simulink model "DWmodel"  (R2025a)
settings: Solver=daessc  StartTime=0.0  StopTime=inf  MaxStep=.5  RelTol=1e-3  AbsTol=1e-3
PreLoadFcn:
  | DWmodel_ini
values from neighbouring files (symbols this model uses):
  basinArea = 0.2    [DWmodel_ini.m]
  heaterPower = 1800    [DWmodel_ini.m]
  inletPipeDia = 0.025    [DWmodel_ini.m]
  inletPipeEffLen = 2    [DWmodel_ini.m]
  lpmLeakageFlow = 0.001    [DWmodel_ini.m]
  machineHeight = 1.5    [DWmodel_ini.m]
  maxBasinLiqLevel = 0.10    (= 0.1)    [DWmodel_ini.m]
  maxBasinLiqTemp = 350    [DWmodel_ini.m]
  minBasinLiqLevel = 0.04    [DWmodel_ini.m]
  minBasinLiqTemp = 305    [DWmodel_ini.m]
  motorPower = 500    [DWmodel_ini.m]
  motorSpeed = 500    [DWmodel_ini.m]
  outletPipeDia = 0.025    [DWmodel_ini.m]
  outletPipeEffLen = 2    [DWmodel_ini.m]
  powerWashCycle = 500    [DWmodel_ini.m]
  pumpOutletDia = 0.025    [DWmodel_ini.m]
libraries: fl_lib x15, nesl_utility x8, simulink x7, SimscapeFluids_lib x3
CloseFcn:
  | try,close(h_DishwasherFaultAnalysis),end
  | clear h_DishwasherFaultAnalysis
  | 
  | clear ambient basinArea machineHeight
  | clear iniBasinLiqLevel maxBasinLiqTemp minBasinLiqTemp
  | clear maxBasinLiqLevel minBasinLiqLevel lpmLeakageFlow
  | clear motorPower motorSpeed heaterPower powerWashCycle
  | clear outletPipeEffLen outletPipeDia inletPipeEffLen inletPipeDia
  | clear pumpOutletDia pumpCapacity pumpHead pumpBrakePower pumpShaftSpeed
  | clear simlog_DishwasherFaultAnalysis tout
Description:
  | Dishwasher Fault Analysis
settings Model: Creator=The MathWorks, Inc.  LastModifiedBy=DR53SF
settings SolverCC: AutoScaleAbsTol=off  MaxConsecutiveMinStep=5  ZeroCrossAlgorithm=Adaptive  AlgebraicLoopSolver=TrustRegion  MaxZcPerStep=1.0
settings DataIOCC: SaveTime=off  ReturnWorkspaceOutputs=off
settings DebuggingCC: IgnoredZcDiagnostic=none  UnconnectedInputMsg=warning  UnconnectedOutputMsg=warning  UnconnectedLineMsg=warning  SymbolicDimsDataTypeCodeGenerationDiagnostic=none
settings ModelReferenceCC: EnableRefExpFcnMdlSchedulingChecks=on
settings SFSimCC: CustomCodeUndefinedFunction=UseInterfaceOnly
settings RTWCC: GPUComputeCapability=3.5  DLArmComputeVersion=19.05
settings SimscapeCC: SimscapeNominalValues="[{\"value\":\"1\",\"unit\":\"A\"},{\"value\":\"1\",\"unit\":\"bar\"},{\"value\":\"1\",\"unit\":\"cm^2\"},{\"value\":\"1\",\"unit\":\"cm^3/s\"},{\"value\":\"1\",\"unit\":\"kJ/kg\"},{\"value\":\"1\",\"unit\":\"kW\"},{\"value\":\"1\",\"unit\":\"l\"},{\"value\":\"1\",\"unit\":\"N\"},{\"value\":\"1\",\"unit\":\"N*m\"},{\"value\":\"1\",\"unit\":\"V\"},{\"value\":\"1e-2\",\"unit\":\"m\"}]"  SimscapeLogType=all  SimscapeLogSimulationStatistics=on  SimscapeLogName=simlog_DishwasherFaultAnalysis  SimscapeLogDataHistory=100000.0

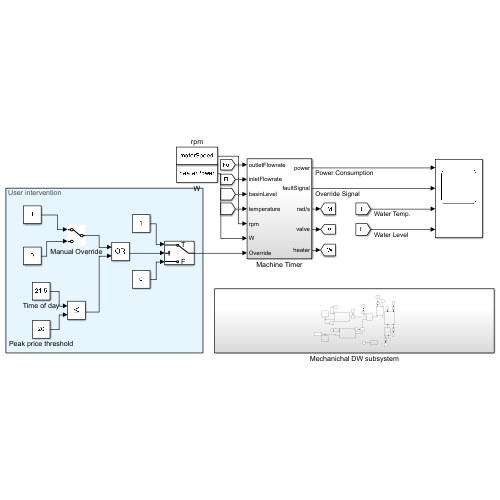
[thumbnail: Simulink's stored preview of the top-level diagram]
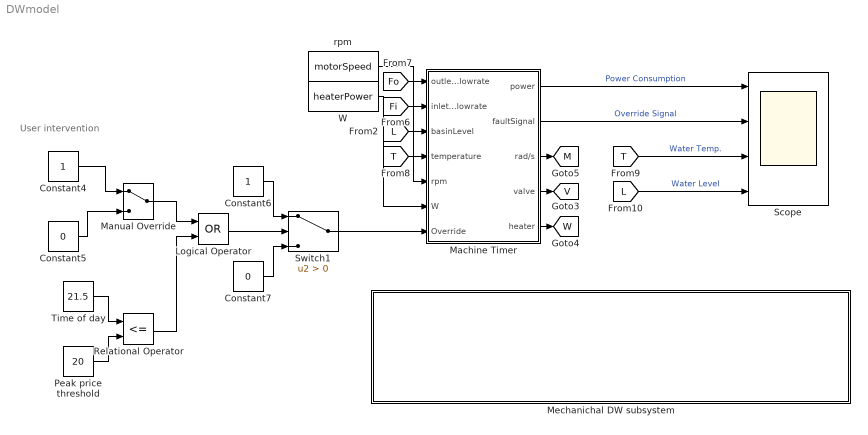
== system DWmodel ==
  note: User intervention
  Constant4 : Constant
  Constant5 : Constant  Value=0
  Constant6 : Constant
  Constant7 : Constant  Value=0
  Logical Operator : Logic  Operator=OR  AllPortsSameDT=off  OutDataTypeStr=boolean
  Machine Timer : Subsystem
  Manual Override : ManualSwitch
  Mechanichal DW subsystem : Subsystem
  Peak price threshold : Constant  Value=20
  Relational Operator : RelationalOperator  Operator=<=  OutDataTypeStr=boolean  RndMeth=Simplest  InputSameDT=off
  Scope : Scope  NumInputPorts=4
      settings: ActiveDisplayYMinimum=-348.81952121815567  ActiveDisplayYMaximum=3139.3756909634017
  Switch1 : Switch  Criteria=u2 > Threshold  SaturateOnIntegerOverflow=off  InputSameDT=off
  Time of day : Constant  Value=21.5
  W : Constant  Value=heaterPower
  rpm : Constant  Value=motorSpeed
  tag scope: M=global, V=global, W=global
  wires:
  [T] -> Scope/3  "Water Temp."
  [L] -> Scope/4  "Water Level"
  [L] -> Machine Timer/3(basinLevel)
  [T] -> Machine Timer/4(temperature)
  Machine Timer/4(valve) -> [V]
  Machine Timer/3(rad/s) -> [M]
  Machine Timer/5(heater) -> [W]
  rpm/1 -> Machine Timer/5(rpm)
  W/1 -> Machine Timer/6(W)
  [Fi] -> Machine Timer/2(inletFlowrate)
  [Fo] -> Machine Timer/1(outletFlowrate)
  Machine Timer/1(power) -> Scope/1  "Power Consumption"
  Machine Timer/2(faultSignal) -> Scope/2  "Override Signal"
  Manual Override/1 -> Logical Operator/1
  Time of day/1 -> Relational Operator/1
  Constant5/1 -> Manual Override/2
  Logical Operator/1 -> Switch1/2
  Constant6/1 -> Switch1/1
  Constant4/1 -> Manual Override/1
  Peak price threshold/1 -> Relational Operator/2
  Constant7/1 -> Switch1/3
  Relational Operator/1 -> Logical Operator/2
  Switch1/1 -> Machine Timer/7(Override)

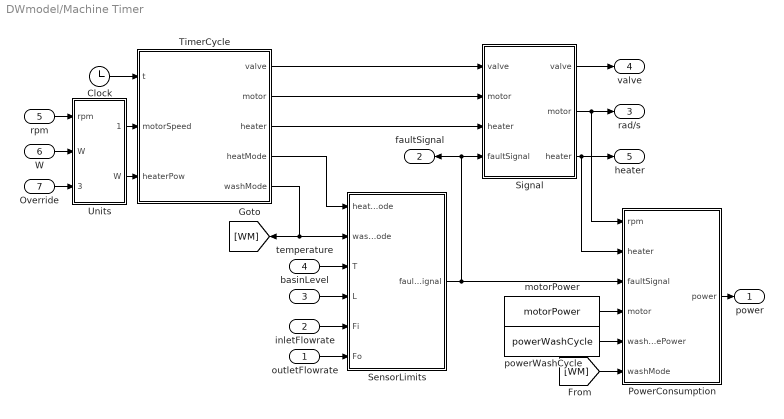
== system DWmodel/Machine Timer ==
  outletFlowrate : Inport
  inletFlowrate : Inport  Port=2
  basinLevel : Inport  Port=3
  temperature : Inport  Port=4
  rpm : Inport  Port=5
  W : Inport  Port=6
  Override : Inport  Port=7
  Clock : Clock
  PowerConsumption : MATLAB Function  TreatAsAtomicUnit=on
  SensorLimits : Subsystem
  Signal : Subsystem
  TimerCycle : MATLAB Function  TreatAsAtomicUnit=on
  Units : Subsystem
  motorPower : Constant  Value=motorPower
  powerWashCycle : Constant  Value=powerWashCycle
  power : Outport
  faultSignal : Outport  Port=2
  rad/s : Outport  Port=3
  valve : Outport  Port=4
  heater : Outport  Port=5
  wires:
  Clock/1 -> TimerCycle/1(t)
  temperature/1 -> SensorLimits/3(T)
  basinLevel/1 -> SensorLimits/4(L)
  TimerCycle/1(valve) -> Signal/1("valve ")
  TimerCycle/2(motor) -> Signal/2("motor ")
  TimerCycle/3(heater) -> Signal/3("heater ")
  Signal/1(valve) -> valve/1
  Signal/2(motor) -> rad/s/1, PowerConsumption/1(rpm)
  Signal/3(heater) -> heater/1, PowerConsumption/2(heater)
  motorPower/1 -> PowerConsumption/4(motor)
  PowerConsumption/1(power) -> power/1
  TimerCycle/4(heatMode) -> SensorLimits/1(heatMode)
  TimerCycle/5(washMode) -> SensorLimits/2(washMode), [WM]
  inletFlowrate/1 -> SensorLimits/5(Fi)
  SensorLimits/1(faultSignal) -> faultSignal/1, Signal/4(faultSignal), PowerConsumption/3(faultSignal)
  powerWashCycle/1 -> PowerConsumption/5(washCyclePower)
  rpm/1 -> Units/1(rpm)
  W/1 -> Units/2(W)
  Override/1 -> Units/3(fault)
  Units/1("rad/s ") -> TimerCycle/2(motorSpeed)
  Units/2("W ") -> TimerCycle/3(heaterPow)
  [WM] -> PowerConsumption/6(washMode)
  outletFlowrate/1 -> SensorLimits/6(Fo)

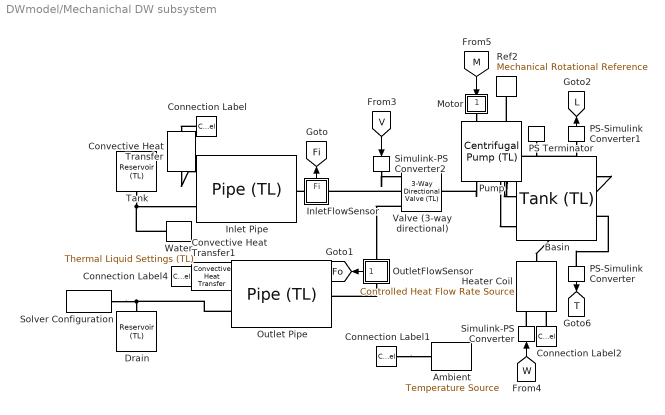
== system DWmodel/Mechanichal DW subsystem ==
  Ambient : fl_lib/Thermal/Thermal Sources/Temperature Source  temperature=ambient K
  Basin : SimscapeFluids_lib/Thermal Liquid/Tanks & Accumulators/Tank (TL)  num_inlet=fluids.thermal_liquid.tanks_accumulators.enum.NumInlet.One  pressure_spec=foundation.enum.pressure_spec.atmospheric  tank_pressure=0.101325 MPa  volume_spec=fluids.thermal_liquid.tanks_accumulators.enum.TankVolumeSpec.Constant  tank_area=basinArea m^2  level_TLU=[0, 3, 5] m  volume_TLU=[0, 4, 6] m^3  inlet_height_A=0 m  inlet_area_A=(pi/4)*pumpOutletDia^2 m^2  inlet_heights_AB=[0, 0] m  inlet_areas_AB=[(pi/4)*inletPipeDia^2, (pi/4)*outletPipeDia^2] m^2  inlet_heights_ABC=[.1, .1, .1] m  inlet_areas_ABC=[.01, .01, .01] m^2  inlet_heights_ABCD=0.1 * ones(1, 4) m  inlet_areas_ABCD=0.01 * ones(1, 4) m^2  inlet_heights_ABCDE=0.1 * ones(1, 5) m  inlet_areas_ABCDE=0.01 * ones(1, 5) m^2  inlet_heights_ABCDEF=0.1 * ones(1, 6) m  inlet_areas_ABCDEF=0.01 * ones(1, 6) m^2  level_check=simscape.enum.assert.action.none  capacity_check=simscape.enum.assert.action.none  max_capacity=basinArea*machineHeight m^3  g=9.81 m/s^2  level_specify=on  level_priority=High  level=iniBasinLiqLevel m  level_nominal_specify=off  level_nominal_value=1  level_nominal_unit=m  volume_specify=off  volume_priority=None  volume=5 m^3  volume_nominal_specify=off  volume_nominal_value=1  volume_nominal_unit=m^3  mass_specify=off  mass_priority=None  mass=5000 kg  mass_nominal_specify=off  mass_nominal_value=1  mass_nominal_unit=kg  T_I_specify=on  T_I_priority=High  T_I=ambient K  T_I_nominal_specify=off  T_I_nominal_value=1  T_I_nominal_unit=K
      settings: InternalSimscapePortConfiguration="{\"Bottom\":[{\"id\":\"H\",\"label\":\"H\",\"type\":\"foundation.thermal.thermal\"},{\"id\":\"T_out\",\"label\":\"T\",\"type\":\"output\"}],\"Left\":[{\"id\":\"A\",\"label\":\"A\",\"type\":\"foundation.thermal_liquid.thermal_liquid\"}],\"Right\":[],\"Top\":[{\"id\":\"V_out\",\"label\":\"V\",\"type\":\"output\"},{\"id\":\"L_out\",\"label\":\"L\",\"type\":\"output\"}]}"
  Connection Label{,1..2,4} (4 alike) : ConnectionLabel  Label=Amb
  Convective Heat Transfer : fl_lib/Thermal/Thermal Elements/Convective Heat Transfer  thermal_type=foundation.enum.constant_variable.constant  area=pi*inletPipeEffLen*inletPipeDia m^2  heat_tr_coeff=20 W/(m^2*K)  min_heat_tr_coeff=1e-3 W/(K*m^2)  T_specify=off  T_priority=None  T=0 K  T_nominal_specify=off  T_nominal_value=1  T_nominal_unit=K  Q_specify=off  Q_priority=None  Q=0 W  Q_nominal_specify=off  Q_nominal_value=1  Q_nominal_unit=W
  Convective Heat Transfer1 : fl_lib/Thermal/Thermal Elements/Convective Heat Transfer  thermal_type=foundation.enum.constant_variable.constant  area=pi*outletPipeEffLen*outletPipeDia m^2  heat_tr_coeff=20 W/(m^2*K)  min_heat_tr_coeff=1e-3 W/(K*m^2)  T_specify=off  T_priority=None  T=0 K  T_nominal_specify=off  T_nominal_value=1  T_nominal_unit=K  Q_specify=off  Q_priority=None  Q=0 W  Q_nominal_specify=off  Q_nominal_value=1  Q_nominal_unit=W
  Drain : fl_lib/Thermal Liquid/Elements/Reservoir (TL)  pressure_spec=foundation.enum.pressure_spec.atmospheric  reservoir_pressure=0.101325 MPa  reservoir_temperature=ambient K  area=(pi/4)*outletPipeDia^2 m^2
  Heater Coil : fl_lib/Thermal/Thermal Sources/Controlled Heat Flow Rate Source
  Inlet Pipe : fl_lib/Thermal Liquid/Elements/Pipe (TL)  length=inletPipeEffLen m  area=(pi/4)*inletPipeDia^2 m^2  Dh=inletPipeDia m  length_add=0.05 m  roughness=15e-6 m  Re_lam=2000  Re_tur=4000  shape_factor=64  Nu_lam=3.66  dynamic_compressibility=simscape.enum.onoff.off  inertia=simscape.enum.onoff.off  p0=0.101325 MPa  T0=ambient K  mdot0=0 kg/s  p_nominal=0.101325 MPa  T_nominal=293.15 K
  InletFlowSensor : Subsystem
      settings: PortSchema="{\"entries\":[{\"content\":{\"sides\":[{\"content\":{\"connectorIds\":[\"LConn1\"]},\"type\":\"ConnectorPlacement.EquallySpacedRectSide\",\"uuid\":\"3c7414fb-f3e3-4bba-af95-6fd6a63baba2\"},{\"content\":{\"connectorIds\":[\"RConn1\"],\"side\":\"RIGHT\"},\"type\":\"ConnectorPlacement.EquallySpacedRectSide\",\"uuid\":\"4a7492a2-ac68-48c8-b5a4-e361ce8e5b30\"},{\"content\":{\"connectorIds\":[\"Out1\"],\"side\":\"TOP\"},\"type\":\"ConnectorPlacement.EquallySpacedRectSide\",\"uuid\":\"4d4f0bbf-9958-4a9a-8aa5-8b025f49d7d3\"}]},\"type\":\"ConnectorPlacement.EquallySpacedConnector\",\"uuid\":\"a70be2c7-f69a-4e84-9929-07b1108312d5\"}],\"packageUris\":[\"http://schema.mathworks.com/mf0/Connector/R2020b\"],\"version\":\"1.0\"}"
  Motor : Subsystem
  Outlet Pipe : fl_lib/Thermal Liquid/Elements/Pipe (TL)  length=outletPipeEffLen m  area=(pi/4)*outletPipeDia^2 m^2  Dh=outletPipeDia m  length_add=0.05 m  roughness=15e-6 m  Re_lam=2000  Re_tur=4000  shape_factor=64  Nu_lam=3.66  dynamic_compressibility=simscape.enum.onoff.off  inertia=simscape.enum.onoff.off  p0=0.101325 MPa  T0=ambient K  mdot0=0 kg/s  p_nominal=0.101325 MPa  T_nominal=293.15 K
  OutletFlowSensor : Subsystem
      settings: PortSchema="{\"entries\":[{\"content\":{\"sides\":[{\"content\":{\"connectorIds\":[\"LConn1\"]},\"type\":\"ConnectorPlacement.EquallySpacedRectSide\",\"uuid\":\"3c7414fb-f3e3-4bba-af95-6fd6a63baba2\"},{\"content\":{\"connectorIds\":[\"RConn1\"],\"side\":\"RIGHT\"},\"type\":\"ConnectorPlacement.EquallySpacedRectSide\",\"uuid\":\"4a7492a2-ac68-48c8-b5a4-e361ce8e5b30\"},{\"content\":{\"connectorIds\":[\"Out1\"],\"side\":\"TOP\"},\"type\":\"ConnectorPlacement.EquallySpacedRectSide\",\"uuid\":\"4d4f0bbf-9958-4a9a-8aa5-8b025f49d7d3\"}]},\"type\":\"ConnectorPlacement.EquallySpacedConnector\",\"uuid\":\"a70be2c7-f69a-4e84-9929-07b1108312d5\"}],\"packageUris\":[\"http://schema.mathworks.com/mf0/Connector/R2020b\"],\"version\":\"1.0\"}"
  PS Terminator : fl_lib/Physical Signals/Sinks/PS Terminator
  PS-Simulink Converter : nesl_utility/PS-Simulink Converter  PhysicalDomain=network_engine_domain  SubClassName=ps_output  LeftPortType=input  RightPortType=output  PseudoPeriodic=off  Frequencies=[]  VectorFormat=inherit  Unit=inherit  AffineConversion=off
  PS-Simulink Converter1 : nesl_utility/PS-Simulink Converter  PhysicalDomain=network_engine_domain  SubClassName=ps_output  LeftPortType=input  RightPortType=output  PseudoPeriodic=off  Frequencies=[]  VectorFormat=inherit  Unit=inherit  AffineConversion=off
  Pump : SimscapeFluids_lib/Thermal Liquid/Pumps & Motors/Centrifugal Pump (TL)  pump_parameterization=fluids.thermal_liquid.pumps_motors.enum.CentrifugalPumpParameterization.Table1D  capacity_ref_nominal=45 lpm  head_ref_nominal=40 m  power_ref_nominal=0.85 kW  head_ref_max=60 m  capacity_ref_max=80 lpm  omega_ref_analytic=1770 rpm  flow_rate_1D_TLU=pumpCapacity lpm  head_1D_TLU=pumpHead m  power_1D_TLU=pumpBrakePower kW  omega_ref_1D=pumpShaftSpeed rpm  rho_ref_1D=998.21 kg/m^3  omega_threshold_factor=1e-2  flow_rate_2D_TLU=[16.67, 23.33, 30, 40, 53.33, 60] lpm  omega_2D_TLU=[2450, 2800, 3150, 3500] rpm  head_2D_TLU=[25, 32.7, 42.5, 50; 24, 31.7, 41, 49; 22.7, 30.5, 39, 47.5; 20, 28, 36, 45; 15.7, 24, 32, 40; 12.5, 21, 29.5, 37.5] m  power_2D_TLU=[.28, .38, .5, .6; .31, .41, .55, .68; .33, .44, .6, .75; .36, .48, .65, .83; .38, .53, .72, .93; .39, .55, .75, .97] kW  rho_ref_2D=998.21 kg/m^3  diameter_ratio=1  mech_orientation=fluids.thermal_liquid.pumps_motors.enum.CentrifugalPumpMechOrientation.Positive  area=(pi/4)*pumpOutletDia^2 m^2  operation_check=simscape.enum.assert.action.none
      settings: InternalSimscapePortConfiguration="{\"Bottom\":[],\"Left\":[{\"id\":\"A\",\"label\":\"A\",\"type\":\"foundation.thermal_liquid.thermal_liquid\"},{\"id\":\"B\",\"label\":\"B\",\"type\":\"foundation.thermal_liquid.thermal_liquid\"}],\"Right\":[{\"id\":\"R\",\"label\":\"R\",\"type\":\"foundation.mechanical.rotational.rotational\"},{\"id\":\"C\",\"label\":\"C\",\"type\":\"foundation.mechanical.rotational.rotational\"}],\"Top\":[]}"
  Ref2 : fl_lib/Mechanical/Rotational Elements/Mechanical Rotational Reference
  Simulink-PS Converter : nesl_utility/Simulink-PS Converter  PhysicalDomain=network_engine_domain  SubClassName=ps_input  LeftPortType=input  RightPortType=output  PseudoPeriodic=off  Frequencies=[]  NoiseDistribution=none  NoiseParameters=[]  Unit=J/s  AffineConversion=off  FilteringAndDerivatives=filter  SimscapeFilterOrder=1  InputFilterTimeConstant=0.001  UdotUserProvided=0
  Simulink-PS Converter2 : nesl_utility/Simulink-PS Converter  PhysicalDomain=network_engine_domain  SubClassName=ps_input  LeftPortType=input  RightPortType=output  PseudoPeriodic=off  Frequencies=[]  NoiseDistribution=none  NoiseParameters=[]  Unit=1  AffineConversion=off  FilteringAndDerivatives=filter  SimscapeFilterOrder=1  InputFilterTimeConstant=0.001  UdotUserProvided=0
  Solver Configuration : nesl_utility/Solver Configuration  PhysicalDomain=network_engine_domain  SubClassName=solver  LeftPortType=input  RightPortType=generic  Tones=[]  Harmonics=[]  SimulateNoise=off  Profile=off  UseLocalSampling=off  EnableSwitchedLinearOptims=on  FrequencyDomain=off  UseCCode=off  RelTol=0.001  AbsTol=1e-06  MinStep=1e-09  ToWorkspace=off  RevertToSquareIcSolve=off  NumHomotopyIterations=100  PhasorMode=off  PhasorModeNumHarmonics=1  ConsistencySolver=NEWTON_XTOL_AFTER_FTOL  IndexReductionMethod=DerivativeReplacement  DoDC=off  ResidualTolerance=1e-9  ConsistencyTolSource=GLOBAL  ConsistencyAbsTol=0.001  ConsistencyRelTol=0.001  ConsistencyTolFactor=0.001  UseLocalSolver=off  LocalSolverChoice=NE_BACKWARD_EULER_ADVANCER  ResolveIndetEquations=on  FunctionEvalNumThread=1  LocalSolverSampleTime=.1  DoFixedCost=off  MaxNonlinIter=50  MaxModeIter=2  ComputeImpulses=off  ImpulseIterations=2  LinearAlgebra=auto  LinearAlgebraNumThread=0  EquationFormulation=NE_TIME_EF  DelaysMemoryBudget=1024  AutomaticFiltering=off  FilteringTimeConstant=0.001  PartitionStorageMethod=AS_NEEDED  PartitionMemoryBudget=1024  PartitionMethod=FAST  MultibodyUseLocalSolver=off  MultibodyLocalSolverChoice=ODE1  MultibodyLocalSolverSampleTime=0.001
  Tank : fl_lib/Thermal Liquid/Elements/Reservoir (TL)  pressure_spec=foundation.enum.pressure_spec.atmospheric  reservoir_pressure=0.101325 MPa  reservoir_temperature=ambient K  area=(pi/4)*inletPipeDia^2 m^2
  Valve (3-way directional) : SimscapeFluids_lib/Thermal Liquid/Valves & Orifices/Directional Control Valves/3-Way Directional Valve (TL)  open_orifices_pos=fluids.thermal_liquid.valves.directional_control_valves.enum.OpenOrifices3Way.PA  open_orifices_neg=fluids.thermal_liquid.valves.directional_control_valves.enum.OpenOrifices3Way.AT  area_spec=fluids.thermal_liquid.valves.directional_control_valves.enum.area_spec.identical  valve_spec=fluids.thermal_liquid.valves.directional_control_valves.enum.ValveSpec.Linear  del_S_max=inletPipeDia/4 m  area_max=(pi/4)*inletPipeDia^2 m^2  del_S_TLU=[0, .002, .004, .007, .017] m  valve_area_TLU=[1e-09, 2.0352e-07, 4.0736e-05, .00011438, .00034356] m^2  del_S_flow_TLU=[0, .002, .004, .007, .017] m  p_diff_TLU=[-.1, .3, .5, .7] MPa  vol_flow_TLU=1e-3 * [1.7e-05, 2e-05, 2.6e-05; .0035, .0045, .0053; .7, .9, 1.06; 1.96, 2.5, 3; 6, 7.7, 9.13] m^3/s  mdot_TLU=[-1e-05, 1.7e-05, 2e-05, 2.6e-05; -.002, .0035, .0045, .0053; -.4, .7, .9, 1.06; -1.13, 1.96, 2.5, 3; -3.45, 6, 7.7, 9.13] kg/s  T_ref_in=293.15 K  p_ref_in=0.101325 MPa  area_leak=1e-10 m^2  Cd=0.7  Re_c=12  smoothing_factor=0.01  pressure_recovery=simscape.enum.onoff.off  area=0.001 m^2  S_max_PA=inletPipeDia m  del_S_max_PA=0.005 m  area_max_PA=1e-4 m^2  del_S_TLU_PA=[0, .002, .004, .007, .017] m  valve_area_TLU_PA=[1e-09, 2.0352e-07, 4.0736e-05, .00011438, .00034356] m^2  del_S_flow_TLU_PA=[0, .002, .004, .007, .017] m  p_diff_TLU_PA=[.3, .5, .7] MPa  vol_flow_TLU_PA=1e-3 * [1.7e-05, 2e-05, 2.6e-05; .0035, .0045, .0053; .7, .9, 1.06; 1.96, 2.5, 3; 6, 7.7, 9.13] m^3/s  mdot_TLU_PA=[1.7e-05, 2e-05, 2.6e-05; .0035, .0045, .0053; .7, .9, 1.06; 1.96, 2.5, 3; 6, 7.7, 9.13] kg/s  S_max_AT=-inletPipeDia m  del_S_max_AT=0.005 m  area_max_AT=1e-4 m^2  del_S_TLU_AT=[0, .002, .004, .007, .017] m  valve_area_TLU_AT=[1e-09, 2.0352e-07, 4.0736e-05, .00011438, .00034356] m^2  del_S_flow_TLU_AT=[0, .002, .004, .007, .017] m  p_diff_TLU_AT=[.3, .5, .7] MPa  vol_flow_TLU_AT=1e-3 * [1.7e-05, 2e-05, 2.6e-05; .0035, .0045, .0053; .7, .9, 1.06; 1.96, 2.5, 3; 6, 7.7, 9.13] m^3/s  mdot_TLU_AT=[1.7e-05, 2e-05, 2.6e-05; .0035, .0045, .0053; .7, .9, 1.06; 1.96, 2.5, 3; 6, 7.7, 9.13] kg/s  S_max_PT=2.5e-3 m  del_S_max_PT=0.005 m  area_max_PT=1e-4 m^2  del_S_TLU_PT=[0, .002, .004, .007, .017] m  valve_area_TLU_PT=[1e-09, 2.0352e-07, 4.0736e-05, .00011438, .00034356] m^2  del_S_flow_TLU_PT=[0, .002, .004, .007, .017] m  p_diff_TLU_PT=[.3, .5, .7] MPa  vol_flow_TLU_PT=1e-3 * [1.7e-05, 2e-05, 2.6e-05; .0035, .0045, .0053; .7, .9, 1.06; 1.96, 2.5, 3; 6, 7.7, 9.13] m^3/s  mdot_TLU_PT=[1.7e-05, 2e-05, 2.6e-05; .0035, .0045, .0053; .7, .9, 1.06; 1.96, 2.5, 3; 6, 7.7, 9.13] kg/s
      settings: InternalSimscapePortConfiguration="{\"Bottom\":[],\"Left\":[{\"id\":\"A\",\"label\":\"A\",\"type\":\"foundation.thermal_liquid.thermal_liquid\"}],\"Right\":[{\"id\":\"S\",\"label\":\"S\",\"type\":\"input\"},{\"id\":\"P\",\"label\":\"P\",\"type\":\"foundation.thermal_liquid.thermal_liquid\"},{\"id\":\"T\",\"label\":\"T\",\"type\":\"foundation.thermal_liquid.thermal_liquid\"}],\"Top\":[]}"
  Water : fl_lib/Thermal Liquid/Utilities/Thermal Liquid Settings (TL)  table_dimensions=foundation.enum.table_dimensions_TL.two_dimensional  T_TLU=[273.1600 : 10 : 373.16]' K  p_TLU=[0.01, 0.1, 5 : 5 : 50] MPa  p_atm=0.101325 MPa  pT_region_flag=foundation.enum.pT_region_TL.min_max  T_min=273.16 K  T_max=363.16 K  p_min=0.05 MPa  p_max=50 MPa  T_min_1D=273.16 K  T_max_1D=363.16 K  p_min_1D=0.05 MPa  p_max_1D=50 MPa  pT_validity_TLU=[1, 1, 1, 1, 1, 1, 1, 1, 1, 1, 1, 1; 1, 1, 1, 1, 1, 1, 1, 1, 1, 1, 1, 1; 1, 1, 1, 1, 1, 1, 1, 1, 1, 1, 1, 1; 1, 1, 1, 1, 1, 1, 1, 1, 1, 1, 1, 1; 1, 1, 1, 1, 1, 1, 1, 1, 1, 1, 1, 1; 0, 1, 1, 1, 1, 1, 1, 1, 1, 1, 1, 1; 0, 1, 1, 1, 1, 1, 1, 1, 1, 1, 1, 1; 0, 1, 1, 1, 1, 1, 1, 1, 1, 1, 1, 1; 0, 1, 1, 1, 1, 1, 1, 1, 1, 1, 1, 1; 0, 1, 1, 1, 1, 1, 1, 1, 1, 1, 1, 1; 0, 0, 1, 1, 1, 1, 1, 1, 1, 1, 1, 1]  properties_range_check=simscape.enum.assert.action.error  rho_parameterization_2D=foundation.enum.rho_parameterization_2D.rho_beta_alpha  rho_parameterization_1D=foundation.enum.rho_parameterization_1D.rho_vector  rho_TLU=[999.7973, 999.8431, 1002.3216, 1004.8218, 1007.293, 1009.7358, 1012.1506, 1014.5379, 1016.8979, 1019.2311, 1021.538, 1023.8188; 999.6579, 999.7009, 1002.0303, 1004.382, 1006.7084, 1009.0101, 1011.2874, 1013.5407, 1015.7703, 1017.9766, 1020.1599, 1022.3206; 998.1632, 998.2045, 1000.4375, 1002.6924, 1004.9239, 1007.1324, 1009.3183, 1011.4819, 1013.6236, 1015.7438, 1017.8428, 1019.921; 995.6057, 995.6458, 997.81864, 1000.0128, 1002.1841, 1004.3332, 1006.4603, 1008.566, 1010.6505, 1012.7144, 1014.758, 1016.7815; 992.1724, 992.2119, 994.35133, 996.5113, 998.6484, 1000.7633, 1002.8563, 1004.928, 1006.9788, 1009.009, 1011.0192, 1013.0097; 988.02, 988.0299, 990.15684, 992.3035, 994.4268, 996.5273, 998.6056, 1000.6622, 1002.6976, 1004.7123, 1006.7067, 1008.6813; 983.18, 983.1901, 985.3217, 987.4721, 989.5983, 991.7008, 993.7803, 995.8374, 997.8726, 999.8864, 1001.8795, 1003.8522; 977.75, 977.7583, 979.9094, 982.0783, 984.2216, 986.34, 988.4343, 990.505, 992.5529, 994.5786, 996.5825, 998.5654; 971.77, 971.7836, 973.96734, 976.1678, 978.3409, 980.4876, 982.6087, 984.7049, 986.7768, 988.8254, 990.8511, 992.8545; 965.26, 965.3023, 967.53107, 969.7753, 971.9901, 974.1764, 976.3354, 978.4676, 980.5741, 982.6556, 984.7129, 986.7465; 958.62, 958.6315, 960.627, 962.9267, 965.1944, 967.4314, 969.6387, 971.8173, 973.9681, 976.0921, 978.19, 980.2628] kg/m^3  beta_TLU=[1.9649, 1.9654, 1.9929, 2.0213, 2.0499, 2.0787, 2.1078, 2.1372, 2.1668, 2.1966, 2.2268, 2.2572; 2.0913, 2.0918, 2.1191, 2.1471, 2.1752, 2.2036, 2.2322, 2.261, 2.2899, 2.3191, 2.3485, 2.3781; 2.1786, 2.1791, 2.2067, 2.235, 2.2634, 2.2919, 2.3206, 2.3494, 2.3784, 2.4075, 2.4367, 2.4661; 2.2332, 2.2337, 2.2619, 2.2908, 2.3197, 2.3487, 2.3778, 2.407, 2.4363, 2.4657, 2.4951, 2.5246; 2.26, 2.2605, 2.2895, 2.3191, 2.3487, 2.3784, 2.4081, 2.4378, 2.4675, 2.4973, 2.5272, 2.5571; 2.2638, 2.2638, 2.2936, 2.324, 2.3544, 2.3848, 2.4151, 2.4455, 2.4758, 2.5062, 2.5365, 2.5669; 2.2472, 2.2472, 2.2779, 2.3092, 2.3403, 2.3715, 2.4025, 2.4336, 2.4646, 2.4955, 2.5264, 2.5573; 2.214, 2.214, 2.2455, 2.2776, 2.3096, 2.3415, 2.3733, 2.405, 2.4367, 2.4683, 2.4998, 2.5313; 2.1668, 2.1668, 2.1992, 2.2321, 2.2649, 2.2976, 2.3301, 2.3626, 2.3949, 2.4272, 2.4593, 2.4914; 2.1081, 2.1081, 2.1413, 2.175, 2.2086, 2.2421, 2.2754, 2.3085, 2.3415, 2.3744, 2.4072, 2.4399; 2.0494, 2.0494, 2.0739, 2.1084, 2.1428, 2.177, 2.211, 2.2449, 2.2786, 2.3121, 2.3455, 2.3788] GPa  alpha_TLU=1e-4 * [-.679, -.676, -.49, -.307, -.13, .041, .206, .365, .519, .668, .811, .949; .878, .881, .998, 1.114, 1.227, 1.337, 1.445, 1.549, 1.651, 1.75, 1.846, 1.939; 2.068, 2.069, 2.141, 2.213, 2.283, 2.352, 2.42, 2.486, 2.551, 2.614, 2.676, 2.736; 3.034, 3.035, 3.074, 3.113, 3.152, 3.191, 3.229, 3.267, 3.305, 3.341, 3.377, 3.413; 3.855, 3.856, 3.87, 3.884, 3.899, 3.914, 3.93, 3.946, 3.961, 3.977, 3.993, 4.009; 4.578, 4.578, 4.572, 4.566, 4.562, 4.558, 4.555, 4.552, 4.55, 4.549, 4.548, 4.547; 5.233, 5.233, 5.209, 5.186, 5.165, 5.144, 5.125, 5.107, 5.09, 5.074, 5.059, 5.045; 5.84, 5.84, 5.801, 5.762, 5.725, 5.691, 5.657, 5.625, 5.595, 5.566, 5.538, 5.512; 6.414, 6.414, 6.36, 6.307, 6.256, 6.208, 6.161, 6.117, 6.074, 6.033, 5.994, 5.956; 6.967, 6.967, 6.898, 6.831, 6.766, 6.705, 6.646, 6.589, 6.535, 6.482, 6.432, 6.384; 7.519, 7.519, 7.423, 7.342, 7.264, 7.189, 7.118, 7.049, 6.983, 6.92, 6.859, 6.8] 1/K  rho_TLU_2=[999.7973, 999.8431, 1002.3216, 1004.8218, 1007.293, 1009.7358, 1012.1506, 1014.5379, 1016.8979, 1019.2311, 1021.538, 1023.8188; 999.6579, 999.7009, 1002.0303, 1004.382, 1006.7084, 1009.0101, 1011.2874, 1013.5407, 1015.7703, 1017.9766, 1020.1599, 1022.3206; 998.1632, 998.2045, 1000.4375, 1002.6924, 1004.9239, 1007.1324, 1009.3183, 1011.4819, 1013.6236, 1015.7438, 1017.8428, 1019.921; 995.6057, 995.6458, 997.81864, 1000.0128, 1002.1841, 1004.3332, 1006.4603, 1008.566, 1010.6505, 1012.7144, 1014.758, 1016.7815; 992.1724, 992.2119, 994.35133, 996.5113, 998.6484, 1000.7633, 1002.8563, 1004.928, 1006.9788, 1009.009, 1011.0192, 1013.0097; 988.02, 988.0299, 990.15684, 992.3035, 994.4268, 996.5273, 998.6056, 1000.6622, 1002.6976, 1004.7123, 1006.7067, 1008.6813; 983.18, 983.1901, 985.3217, 987.4721, 989.5983, 991.7008, 993.7803, 995.8374, 997.8726, 999.8864, 1001.8795, 1003.8522; 977.75, 977.7583, 979.9094, 982.0783, 984.2216, 986.34, 988.4343, 990.505, 992.5529, 994.5786, 996.5825, 998.5654; 971.77, 971.7836, 973.96734, 976.1678, 978.3409, 980.4876, 982.6087, 984.7049, 986.7768, 988.8254, 990.8511, 992.8545; 965.26, 965.3023, 967.53107, 969.7753, 971.9901, 974.1764, 976.3354, 978.4676, 980.5741, 982.6556, 984.7129, 986.7465; 958.62, 958.6315, 960.627, 962.9267, 965.1944, 967.4314, 969.6387, 971.8173, 973.9681, 976.0921, 978.19, 980.2628] kg/m^3  rho_ref_3=998.21 kg/m^3  T_ref_3=293.16 K  p_ref_3=0.101325 MPa  beta_const_3=2.1791 GPa  alpha_const_3=2.0691e-4 1/K  rho_TLU_4=[999.84; 999.7; 998.2; 995.65; 992.21; 988.03; 983.19; 977.76; 971.78; 965.3; 958.8] kg/m^3  beta_const_4=2.1791 GPa  p_ref_4=0.101325 MPa  rho_ref_5=998.21 kg/m^3  T_ref_5=293.16 K  p_ref_5=0.101325 MPa  beta_const_5=2.1791 GPa  alpha_const_5=2.0691e-4 1/K  u_parameterization_2D=foundation.enum.u_parameterization_2D.u_cp  u_parameterization_1D=foundation.enum.u_parameterization_1D.u  u_TLU=[.0002, .0018, .086, .1588, .219, .267, .3034, .3288, .3436, .3483, .3435, .3294; 42.062, 42.06, 41.935, 41.804, 41.668, 41.527, 41.382, 41.233, 41.081, 40.924, 40.763, 40.599; 83.953, 83.948, 83.651, 83.349, 83.049, 82.749, 82.451, 82.153, 81.856, 81.56, 81.265, 80.971; 125.77, 125.76, 125.31, 124.86, 124.41, 123.97, 123.53, 123.1, 122.68, 122.25, 121.84, 121.42; 167.57, 167.56, 166.96, 166.37, 165.79, 165.21, 164.65, 164.09, 163.54, 163, 162.46, 161.94; 209.36, 209.36, 208.63, 207.9, 207.19, 206.48, 205.79, 205.11, 204.45, 203.79, 203.14, 202.5; 251.19, 251.19, 250.33, 249.47, 248.62, 247.79, 246.98, 246.18, 245.39, 244.62, 243.86, 243.12; 293.06, 293.06, 292.07, 291.07, 290.1, 289.14, 288.2, 287.28, 286.38, 285.49, 284.62, 283.77; 334.99, 334.99, 333.86, 332.73, 331.63, 330.54, 329.48, 328.44, 327.41, 326.41, 325.43, 324.46; 377, 377, 375.73, 374.46, 373.22, 372, 370.81, 369.64, 368.5, 367.38, 366.27, 365.19; 419.01, 419.01, 417.69, 416.27, 414.89, 413.54, 412.21, 410.91, 409.64, 408.4, 407.17, 405.98] kJ/kg  cp_TLU=[4.2199, 4.2194, 4.1957, 4.1726, 4.1508, 4.13, 4.1103, 4.0916, 4.0738, 4.0569, 4.0408, 4.0254; 4.1955, 4.1951, 4.1769, 4.1592, 4.1422, 4.1259, 4.1103, 4.0954, 4.0812, 4.0676, 4.0545, 4.0421; 4.1843, 4.184, 4.169, 4.1543, 4.1401, 4.1264, 4.1133, 4.1007, 4.0885, 4.0768, 4.0656, 4.0548; 4.1801, 4.1798, 4.1667, 4.1538, 4.1413, 4.1293, 4.1177, 4.1064, 4.0956, 4.0851, 4.075, 4.0653; 4.1796, 4.1794, 4.1675, 4.1558, 4.1444, 4.1334, 4.1227, 4.1123, 4.1023, 4.0926, 4.0832, 4.0741; 4.1813, 4.1813, 4.1702, 4.1592, 4.1484, 4.138, 4.1279, 4.1181, 4.1086, 4.0993, 4.0903, 4.0816; 4.185, 4.185, 4.1742, 4.1636, 4.1532, 4.1432, 4.1334, 4.1239, 4.1146, 4.1056, 4.0969, 4.0884; 4.1901, 4.1901, 4.1795, 4.169, 4.1588, 4.1489, 4.1393, 4.1299, 4.1207, 4.1118, 4.1032, 4.0947; 4.1968, 4.1968, 4.1862, 4.1757, 4.1655, 4.1555, 4.1458, 4.1364, 4.1273, 4.1183, 4.1096, 4.1012; 4.2052, 4.2052, 4.1944, 4.1837, 4.1733, 4.1632, 4.1534, 4.1438, 4.1345, 4.1255, 4.1166, 4.108; 4.2136, 4.2136, 4.2045, 4.1935, 4.1828, 4.1724, 4.1623, 4.1524, 4.1429, 4.1335, 4.1245, 4.1157] kJ/(K*kg)  u_TLU_2=[.0002, .0018, .086, .1588, .219, .267, .3034, .3288, .3436, .3483, .3435, .3294; 42.062, 42.06, 41.935, 41.804, 41.668, 41.527, 41.382, 41.233, 41.081, 40.924, 40.763, 40.599; 83.953, 83.948, 83.651, 83.349, 83.049, 82.749, 82.451, 82.153, 81.856, 81.56, 81.265, 80.971; 125.77, 125.76, 125.31, 124.86, 124.41, 123.97, 123.53, 123.1, 122.68, 122.25, 121.84, 121.42; 167.57, 167.56, 166.96, 166.37, 165.79, 165.21, 164.65, 164.09, 163.54, 163, 162.46, 161.94; 209.36, 209.36, 208.63, 207.9, 207.19, 206.48, 205.79, 205.11, 204.45, 203.79, 203.14, 202.5; 251.19, 251.19, 250.33, 249.47, 248.62, 247.79, 246.98, 246.18, 245.39, 244.62, 243.86, 243.12; 293.06, 293.06, 292.07, 291.07, 290.1, 289.14, 288.2, 287.28, 286.38, 285.49, 284.62, 283.77; 334.99, 334.99, 333.86, 332.73, 331.63, 330.54, 329.48, 328.44, 327.41, 326.41, 325.43, 324.46; 377, 377, 375.73, 374.46, 373.22, 372, 370.81, 369.64, 368.5, 367.38, 366.27, 365.19; 419.01, 419.01, 417.69, 416.27, 414.89, 413.54, 412.21, 410.91, 409.64, 408.4, 407.17, 405.98] kJ/kg  cp_TLU_3=[4.2199, 4.2194, 4.1957, 4.1726, 4.1508, 4.13, 4.1103, 4.0916, 4.0738, 4.0569, 4.0408, 4.0254; 4.1955, 4.1951, 4.1769, 4.1592, 4.1422, 4.1259, 4.1103, 4.0954, 4.0812, 4.0676, 4.0545, 4.0421; 4.1843, 4.184, 4.169, 4.1543, 4.1401, 4.1264, 4.1133, 4.1007, 4.0885, 4.0768, 4.0656, 4.0548; 4.1801, 4.1798, 4.1667, 4.1538, 4.1413, 4.1293, 4.1177, 4.1064, 4.0956, 4.0851, 4.075, 4.0653; 4.1796, 4.1794, 4.1675, 4.1558, 4.1444, 4.1334, 4.1227, 4.1123, 4.1023, 4.0926, 4.0832, 4.0741; 4.1813, 4.1813, 4.1702, 4.1592, 4.1484, 4.138, 4.1279, 4.1181, 4.1086, 4.0993, 4.0903, 4.0816; 4.185, 4.185, 4.1742, 4.1636, 4.1532, 4.1432, 4.1334, 4.1239, 4.1146, 4.1056, 4.0969, 4.0884; 4.1901, 4.1901, 4.1795, 4.169, 4.1588, 4.1489, 4.1393, 4.1299, 4.1207, 4.1118, 4.1032, 4.0947; 4.1968, 4.1968, 4.1862, 4.1757, 4.1655, 4.1555, 4.1458, 4.1364, 4.1273, 4.1183, 4.1096, 4.1012; 4.2052, 4.2052, 4.1944, 4.1837, 4.1733, 4.1632, 4.1534, 4.1438, 4.1345, 4.1255, 4.1166, 4.108; 4.2136, 4.2136, 4.2045, 4.1935, 4.1828, 4.1724, 4.1623, 4.1524, 4.1429, 4.1335, 4.1245, 4.1157] kJ/(K*kg)  u_TLU_4=[.0018; 42.06; 83.948; 125.76; 167.56; 209.36; 251.19; 293.06; 334.99; 377; 418.01] kJ/kg  cp_TLU_5=[4.2199; 4.1955; 4.1843; 4.1801; 4.1796; 4.1813; 4.185; 4.1901; 4.1968; 4.2052; 4.2136] kJ/(K*kg)  nu_TLU=[1.7917, 1.7914, 1.7763, 1.7615, 1.7473, 1.7338, 1.7208, 1.7085, 1.6967, 1.6854, 1.6747, 1.6645; 1.3061, 1.3059, 1.2986, 1.2914, 1.2845, 1.2779, 1.2716, 1.2656, 1.2598, 1.2543, 1.2491, 1.2441; 1.0032, 1.0032, .9995, .9959, .9924, .9891, .9859, .9829, .9801, .9774, .9748, .9724; .8006, .8005, .7987, .797, .7953, .7937, .7922, .7908, .7894, .7881, .787, .7859; .6577, .6577, .657, .6562, .6555, .6548, .6543, .6537, .6532, .6528, .6523, .652; .553, .553, .5529, .5527, .5526, .5525, .5524, .5524, .5524, .5524, .5524, .5525; .4739, .4739, .4741, .4743, .4745, .4747, .475, .4753, .4755, .4758, .4762, .4765; .4127, .4127, .4131, .4135, .4139, .4143, .4148, .4152, .4157, .4162, .4167, .4172; .3643, .3643, .3648, .3654, .3659, .3665, .367, .3676, .3682, .3688, .3694, .37; .3254, .3254, .3261, .3267, .3273, .328, .3286, .3293, .3299, .3306, .3312, .3319; .2866, .2866, .2945, .2952, .2959, .2965, .2972, .2979, .2986, .2993, .3, .3007] mm^2/s  nu_TLU_2=[1.7917; 1.3061; 1.0032; .8006; .6577; .553; .4739; .4127; .3643; .3254; .2866] mm^2/s  k_TLU=[561.04, 561.09, 563.8, 566.56, 569.32, 572.08, 574.82, 577.54, 580.24, 582.92, 585.57, 588.18; 580.02, 580.07, 582.45, 584.88, 587.32, 589.75, 592.18, 594.61, 597.02, 599.42, 601.8, 604.16; 598.44, 598.48, 600.73, 603.03, 605.33, 607.64, 609.94, 612.24, 614.54, 616.82, 619.1, 621.36; 615.48, 615.52, 617.73, 620, 622.26, 624.54, 626.81, 629.07, 631.34, 633.6, 635.85, 638.09; 630.6, 630.64, 632.87, 635.15, 637.44, 639.72, 642.01, 644.29, 646.57, 648.84, 651.11, 653.36; 643.61, 643.61, 645.88, 648.21, 650.53, 652.86, 655.18, 657.51, 659.82, 662.14, 664.44, 666.74; 654.39, 654.39, 656.73, 659.12, 661.5, 663.89, 666.27, 668.65, 671.02, 673.38, 675.74, 678.09; 663.13, 663.13, 665.54, 668, 670.46, 672.91, 675.36, 677.8, 680.24, 682.67, 685.09, 687.5; 670.02, 670.02, 672.51, 675.05, 677.59, 680.12, 682.64, 685.16, 687.67, 690.17, 692.66, 695.14; 675.27, 675.27, 677.85, 680.48, 683.11, 685.73, 688.34, 690.94, 693.53, 696.11, 698.68, 701.24; 680.52, 680.52, 681.77, 684.5, 687.22, 689.94, 692.64, 695.34, 698.02, 700.69, 703.35, 706] mW/(K*m)  k_TLU_2=[561.04; 580.02; 598.44; 615.48; 630.6; 643.61; 654.39; 663.13; 670.02; 675.27; 680.52] mW/(K*m)
  tag scope: Fi=global, Fo=global, L=global, T=global
  wires:
  InletFlowSensor/1(Fi) -> [Fi]
  OutletFlowSensor/1(Fo) -> [Fo]
  [M] -> Motor/1(" ")
  PS-Simulink Converter/1 -> [T]
  [V] -> Simulink-PS Converter2/1
  [W] -> Simulink-PS Converter/1
  PS-Simulink Converter1/1 -> [L]
  connections:
  Tank/LConn1 -- Water/RConn1 -- Inlet Pipe/LConn1
  PS Terminator/LConn1 -- Basin/LConn2
  Motor/RConn1 -- Pump/RConn1
  PS-Simulink Converter1/LConn1 -- Basin/LConn3
  Connection Label/LConn1 -- Convective Heat Transfer/RConn1
  Outlet Pipe/LConn1 -- Solver Configuration/RConn1 -- Drain/LConn1
  Pump/RConn2 -- Ref2/LConn1
  Valve (3-way directional)/RConn3 -- OutletFlowSensor/LConn1
  Simulink-PS Converter/RConn1 -- Heater Coil/RConn1
  Connection Label2/LConn1 -- Heater Coil/RConn2
  Pump/LConn1 -- Valve (3-way directional)/LConn1
  Convective Heat Transfer1/LConn1 -- Outlet Pipe/LConn2
  Convective Heat Transfer/LConn1 -- Inlet Pipe/LConn2
  Pump/LConn2 -- Basin/LConn1
  InletFlowSensor/LConn1 -- Inlet Pipe/RConn1
  Basin/RConn1 -- Heater Coil/LConn1
  Connection Label4/LConn1 -- Convective Heat Transfer1/RConn1
  Valve (3-way directional)/RConn2 -- InletFlowSensor/RConn1
  PS-Simulink Converter/LConn1 -- Basin/RConn2
  OutletFlowSensor/RConn1 -- Outlet Pipe/RConn1
  Simulink-PS Converter2/RConn1 -- Valve (3-way directional)/RConn1
  Connection Label1/LConn1 -- Ambient/LConn1

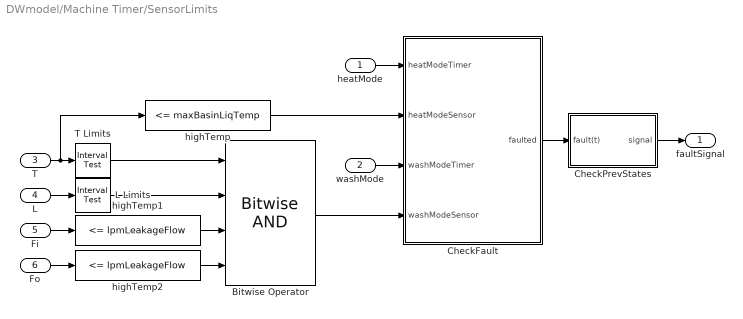
== system DWmodel/Machine Timer/SensorLimits ==
  heatMode : Inport
  washMode : Inport  Port=2
  T : Inport  Port=3
  L : Inport  Port=4
  Fi : Inport  Port=5
  Fo : Inport  Port=6
  Bitwise Operator : simulink/Logic and Bit Operations/Bitwise Operator  logicop=AND  UseBitMask=off  NumInputPorts=4  BitMask=bin2dec('11011001')  BitMaskRealWorld=Stored Integer
  CheckFault : MATLAB Function  TreatAsAtomicUnit=on
  CheckPrevStates : Subsystem
  L Limits : simulink/Logic and Bit Operations/Interval Test  IntervalClosedRight=on  uplimit=maxBasinLiqLevel  IntervalClosedLeft=on  lowlimit=minBasinLiqLevel  OutDataTypeStr=boolean
  T Limits : simulink/Logic and Bit Operations/Interval Test  IntervalClosedRight=on  uplimit=maxBasinLiqTemp  IntervalClosedLeft=on  lowlimit=minBasinLiqTemp  OutDataTypeStr=boolean
  highTemp : simulink/Logic and Bit Operations/Compare To Constant  relop=<=  const=maxBasinLiqTemp  OutDataTypeStr=boolean
  highTemp1 : simulink/Logic and Bit Operations/Compare To Constant  relop=<=  const=lpmLeakageFlow  OutDataTypeStr=boolean
  highTemp2 : simulink/Logic and Bit Operations/Compare To Constant  relop=<=  const=lpmLeakageFlow  OutDataTypeStr=boolean
  faultSignal : Outport
  wires:
  T Limits/1 -> Bitwise Operator/1
  L Limits/1 -> Bitwise Operator/2
  L/1 -> L Limits/1
  T/1 -> highTemp/1, T Limits/1
  heatMode/1 -> CheckFault/1(heatModeTimer)
  Bitwise Operator/1 -> CheckFault/4(washModeSensor)
  highTemp/1 -> CheckFault/2(heatModeSensor)
  washMode/1 -> CheckFault/3(washModeTimer)
  Fi/1 -> highTemp1/1
  highTemp1/1 -> Bitwise Operator/3
  highTemp2/1 -> Bitwise Operator/4
  Fo/1 -> highTemp2/1
  CheckFault/1(faulted) -> CheckPrevStates/1(fault(t))
  CheckPrevStates/1(signal) -> faultSignal/1

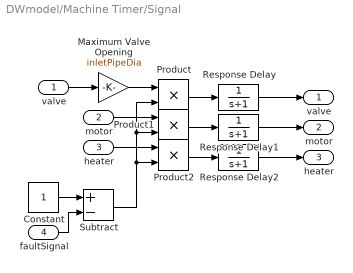
== system DWmodel/Machine Timer/Signal ==
  "valve " : Inport
  "motor " : Inport  Port=2
  "heater " : Inport  Port=3
  faultSignal : Inport  Port=4
  Constant : Constant
  Maximum Valve Opening : Gain  Gain=inletPipeDia
  Product : Product
  Product1 : Product
  Product2 : Product
  Response Delay : TransferFcn  Denominator=[1 1]
  Response Delay1 : TransferFcn  Denominator=[1 1]
  Response Delay2 : TransferFcn  Denominator=[1 1]
  Subtract : Sum  Inputs=+-
  valve : Outport
  motor : Outport  Port=2
  heater : Outport  Port=3
  wires:
  Response Delay1/1 -> motor/1
  Product1/1 -> Response Delay1/1
  Product2/1 -> Response Delay2/1
  Response Delay2/1 -> heater/1
  Response Delay/1 -> valve/1
  "heater "/1 -> Product2/1
  "motor "/1 -> Product1/1
  Product/1 -> Response Delay/1
  Constant/1 -> Subtract/1
  faultSignal/1 -> Subtract/2
  Subtract/1 -> Product2/2, Product1/2, Product/2
  Maximum Valve Opening/1 -> Product/1
  "valve "/1 -> Maximum Valve Opening/1

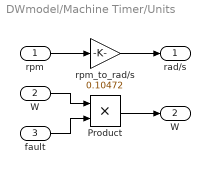
== system DWmodel/Machine Timer/Units ==
  rpm : Inport
  W : Inport  Port=2
  fault : Inport  Port=3
  Product : Product
  rpm_to_rad/s : Gain  Gain=0.10472
  "rad/s " : Outport
  "W " : Outport  Port=2
  wires:
  rpm_to_rad/s/1 -> "rad/s "/1
  rpm/1 -> rpm_to_rad/s/1
  W/1 -> Product/1
  fault/1 -> Product/2
  Product/1 -> "W "/1

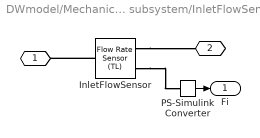
== system DWmodel/Mechanichal DW subsystem/InletFlowSensor ==
  InletFlowSensor : fl_lib/Thermal Liquid/Sensors/Flow Rate Sensor (TL)  mass_flow_measure=false  volumetric_flow_measure=true  energy_flow_measure=false
      settings: InternalSimscapePortConfiguration="{\"Bottom\":[],\"Left\":[{\"id\":\"A\",\"label\":\"A\",\"type\":\"foundation.thermal_liquid.thermal_liquid\"}],\"Right\":[{\"id\":\"B\",\"label\":\"B\",\"type\":\"foundation.thermal_liquid.thermal_liquid\"},{\"id\":\"V\",\"label\":\"V\",\"type\":\"output\"}],\"Top\":[]}"
  PS-Simulink Converter : nesl_utility/PS-Simulink Converter  PhysicalDomain=network_engine_domain  SubClassName=ps_output  LeftPortType=input  RightPortType=output  PseudoPeriodic=off  Frequencies=[]  VectorFormat=inherit  Unit=inherit  AffineConversion=off
  " " : PMIOPort  Side=Left
  "  " : PMIOPort  Port=2  Side=Right
  Fi : Outport
  wires:
  PS-Simulink Converter/1 -> Fi/1
  connections:
  InletFlowSensor/RConn1 -- "  "/RConn1
  InletFlowSensor/LConn1 -- " "/RConn1
  InletFlowSensor/RConn2 -- PS-Simulink Converter/LConn1

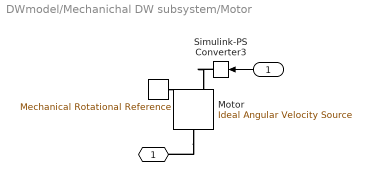
== system DWmodel/Mechanichal DW subsystem/Motor ==
  " " : Inport
  "      " : fl_lib/Mechanical/Rotational Elements/Mechanical Rotational Reference
  Motor : fl_lib/Mechanical/Mechanical Sources/Ideal Angular Velocity Source
  Simulink-PS Converter3 : nesl_utility/Simulink-PS Converter  PhysicalDomain=network_engine_domain  SubClassName=ps_input  LeftPortType=input  RightPortType=output  PseudoPeriodic=off  Frequencies=[]  NoiseDistribution=none  NoiseParameters=[]  Unit=rad/s  AffineConversion=off  FilteringAndDerivatives=filter  SimscapeFilterOrder=1  InputFilterTimeConstant=0.001  UdotUserProvided=0
  "  " : PMIOPort  Side=Right
  wires:
  " "/1 -> Simulink-PS Converter3/1
  connections:
  "      "/LConn1 -- Motor/RConn2
  Simulink-PS Converter3/RConn1 -- Motor/RConn1
  Motor/LConn1 -- "  "/RConn1

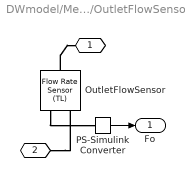
== system DWmodel/Mechanichal DW subsystem/OutletFlowSensor ==
  OutletFlowSensor : fl_lib/Thermal Liquid/Sensors/Flow Rate Sensor (TL)  mass_flow_measure=false  volumetric_flow_measure=true  energy_flow_measure=false
      settings: InternalSimscapePortConfiguration="{\"Bottom\":[],\"Left\":[{\"id\":\"A\",\"label\":\"A\",\"type\":\"foundation.thermal_liquid.thermal_liquid\"}],\"Right\":[{\"id\":\"B\",\"label\":\"B\",\"type\":\"foundation.thermal_liquid.thermal_liquid\"},{\"id\":\"V\",\"label\":\"V\",\"type\":\"output\"}],\"Top\":[]}"
  PS-Simulink Converter : nesl_utility/PS-Simulink Converter  PhysicalDomain=network_engine_domain  SubClassName=ps_output  LeftPortType=input  RightPortType=output  PseudoPeriodic=off  Frequencies=[]  VectorFormat=inherit  Unit=inherit  AffineConversion=off
  " " : PMIOPort  Side=Left
  "  " : PMIOPort  Port=2  Side=Right
  Fo : Outport
  wires:
  PS-Simulink Converter/1 -> Fo/1
  connections:
  OutletFlowSensor/LConn1 -- " "/RConn1
  "  "/RConn1 -- OutletFlowSensor/RConn1
  OutletFlowSensor/RConn2 -- PS-Simulink Converter/LConn1

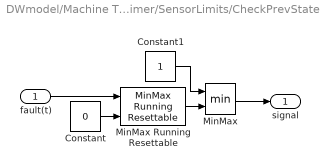
== system DWmodel/Machine Timer/SensorLimits/CheckPrevStates ==
  fault(t) : Inport
  Constant : Constant  Value=0
  Constant1 : Constant
  MinMax : MinMax  Inputs=2
  MinMax Running Resettable : simulink/Math Operations/MinMax Running Resettable  Function=max  vinit=0
  signal : Outport
  wires:
  MinMax Running Resettable/1 -> MinMax/2
  MinMax/1 -> signal/1
  Constant1/1 -> MinMax/1
  fault(t)/1 -> MinMax Running Resettable/1
  Constant/1 -> MinMax Running Resettable/2

== matlab function DWmodel/Machine Timer/PowerConsumption ==
  data: rpm input; heater input; faultSignal input; power output; motor input; washCyclePower input; washMode input
function power = POW(rpm,heater,faultSignal,motor,washCyclePower,washMode)
    % This block calculates power consumption due to heating element, wash
    % cycle and fluid pumping
    % 
    % rpm           : motor rpm
    % heater        : power consumption by heating element [W]
    % washCyclePower: power consumption during wash cycle [W]
    % motor         : pump power consumption [W]
    %
    if rpm==0
        motorPower=0;
    else
        motorPower=motor;
    end
    if washMode
        power=heater+motorPower+washCyclePower*(1-faultSignal);
    else
        power=heater+motorPower;
    end
end

== matlab function DWmodel/Machine Timer/TimerCycle ==
  data: t input; valve output; motor output; heater output; heatMode output; motorSpeed input; heaterPow input; washMode output
function [valve,motor,heater,heatMode,washMode]  = Timer(t,motorSpeed,heaterPow)
    % This block defines a typical timer based wash cycle
    % 
    oneMin=60;                % internal variable, one minute [s]
    fillMode=false;           % fill or drain operation
    heatMode=false;           % heating operation
    washMode=false;           % washing or rinse operation
    valve=0;                  % valves are closed
    motor=0;                  % motor is not operating
    heater=0;                 % heater is switched off
    % Set 'inletOutletParam' to  1 for Inlet Open
    %                        to -1 for Outlet Open
    %                        to  0 for Inlet and Outlet closed
    if t<=2*oneMin
        % Fill
        inletOutletParam=1;
        heater=0;
        fillMode=true;
    elseif t>2*oneMin && t<=4*oneMin
        % pre-Rinse
        inletOutletParam=0;
        heater=0;
    elseif t>4*oneMin && t<=10*oneMin
        % Heat
        inletOutletParam=0;
        heater=heaterPow;
        heatMode=true;
    elseif t>10*oneMin && t<30*oneMin
        % Wash
        inletOutletParam=0;
        heater=0;
        washMode=true;
    elseif t>30*oneMin && t<=32*oneMin
        % Drain
        inletOutletParam=-1;
        heater=0;
        fillMode=true;
    elseif t>32*oneMin && t<=34*oneMin
        % Fill again
        inletOutletParam=1;
        heater=heaterPow;
        fillMode=true;heatMode=true;
    elseif t>34*oneMin && t<=40*oneMin 
        % Heat
        heater=heaterPow;
        heatMode=true;
        inletOutletParam=0;
    elseif t>40*oneMin && t<=60*oneMin 
        % Rinse and clean
        inletOutletParam=0;
        heater=0;
        washMode=true;
    elseif t>60*oneMin && t<=62*oneMin 
        % Drain
        inletOutletParam=-1;
        heater=0;
        fillMode=true;
    else
        % Dry & end
        inletOutletParam=0;
        heater=0;
    end
    valve=inletOutletParam;
    motor=inletOutletParam*motorSpeed;
end

== matlab function DWmodel/Machine Timer/SensorLimits/CheckFault ==
  data: heatModeTimer input; faulted output; heatModeSensor input; washModeTimer input; washModeSensor input
function faulted = faultDetect(heatModeTimer,heatModeSensor,washModeTimer,washModeSensor)
    % heatModeTimer : Heat Mode (true/false) as per TimerCycle block
    % washModeTimer : Wash Mode (true/false) as per TimerCycle block
    % heatModeSensor: Heat Mode can be safely operated (true/false)
    % washModeSensor: Wash Mode can be safely operated (true/false)
    %
    faulted=0;
    if heatModeTimer==true && heatModeSensor==false
        faulted=1;
    end
    if washModeTimer==true && washModeSensor==false
        faulted=1;
    end
end
